simulink model "HybridFEMModel"  (Simulink 7.0)
settings: Solver=FixedStepDiscrete  SolverMode=SingleTasking  StartTime=0.0  StopTime=RunningTime  FixedStep=SampleRate  RelTol=1e-3
undefined symbols (not defined in the file): Alpham, DiscIntNeverNeededParam, Elements, gamma1, gamma2, sample, SampleRate
libraries: simulink x6
(part 3 of 4)

== system HybridFEMModel/Quad Ramp Gen AIC/inverse compensator ==
  note: dp
  note: d(alpha)
  note: dc
  In1 : Inport  OutDataType=sfix(16)  OutScaling=2^0
  In2 : Inport  Port=2  OutDataType=sfix(16)  OutScaling=2^0
  Discrete Transfer Fcn : DiscreteTransferFcn  Numerator=[1 -1]  Denominator=[1 0]  SampleTime=sample
  Product : Product  OutDataType=sfix(16)  OutScaling=2^0  RndMeth=Zero
  Scope : Scope
  Sum2 : Sum  Inputs=|++  OutDataType=sfix(16)  OutScaling=2^0
  Sum5 : Sum  Inputs=|++  OutDataType=sfix(16)  OutScaling=2^0
  Unit Delay : UnitDelay  SampleTime=sample
  alpham : Constant  Value=Alpham  OutDataType=sfix(16)  OutScaling=2^0
  Out1 : Outport  OutDataType=sfix(16)  OutScaling=2^0
  wires:
  Sum2/1 -> Out1/1
  Product/1 -> Sum2/2
  Unit Delay/1 -> Sum2/1
  Sum5/1 -> Scope/1, Product/2
  Discrete Transfer Fcn/1 -> Product/1
  alpham/1 -> Sum5/2
  In2/1 -> Sum5/1
  In1/1 -> Unit Delay/1, Discrete Transfer Fcn/1

== system HybridFEMModel/Linear AIC/Tracking Indicator/A ==
  note: TI
  note: dm
  note: dc
  In1 : Inport  OutDataType=sfix(16)  OutScaling=2^0
  In2 : Inport  Port=2  OutDataType=sfix(16)  OutScaling=2^0
  Gain : Gain  Gain=0.5  ParameterDataType=sfix(16)  ParameterScaling=2^0  OutDataType=sfix(16)  OutScaling=2^0
  Product1 : Product  OutDataType=sfix(16)  OutScaling=2^0  RndMeth=Zero
  Sum2 : Sum  Inputs=|++  OutDataType=sfix(16)  OutScaling=2^0
  Sum3 : Sum  Inputs=|+-  OutDataType=sfix(16)  OutScaling=2^0
  Unit Delay : UnitDelay  SampleTime=sample
  Unit Delay1 : UnitDelay  SampleTime=sample
  accumulation : DiscreteTransferFcn  Numerator=[1 0]  Denominator=[1 -1]  SampleTime=sample
  Out1 : Outport  OutDataType=sfix(16)  OutScaling=2^0
  wires:
  accumulation/1 -> Out1/1
  Gain/1 -> accumulation/1
  Product1/1 -> Gain/1
  Sum3/1 -> Product1/2
  Sum2/1 -> Product1/1
  Unit Delay1/1 -> Sum3/2
  Unit Delay/1 -> Sum2/1
  In2/1 -> Unit Delay1/1, Sum3/1
  In1/1 -> Sum2/2, Unit Delay/1

== system HybridFEMModel/Linear AIC/Tracking Indicator/TA ==
  note: TI
  note: dc
  note: dm
  In1 : Inport  OutDataType=sfix(16)  OutScaling=2^0
  In2 : Inport  Port=2  OutDataType=sfix(16)  OutScaling=2^0
  Gain : Gain  Gain=0.5  ParameterDataType=sfix(16)  ParameterScaling=2^0  OutDataType=sfix(16)  OutScaling=2^0
  Product1 : Product  OutDataType=sfix(16)  OutScaling=2^0  RndMeth=Zero
  Sum2 : Sum  Inputs=|++  OutDataType=sfix(16)  OutScaling=2^0
  Sum3 : Sum  Inputs=|+-  OutDataType=sfix(16)  OutScaling=2^0
  Unit Delay : UnitDelay  SampleTime=sample
  Unit Delay1 : UnitDelay  SampleTime=sample
  accumulation : DiscreteTransferFcn  Numerator=[1 0]  Denominator=[1 -1]  SampleTime=sample
  Out1 : Outport  OutDataType=sfix(16)  OutScaling=2^0
  wires:
  accumulation/1 -> Out1/1
  Gain/1 -> accumulation/1
  Product1/1 -> Gain/1
  Sum3/1 -> Product1/2
  Sum2/1 -> Product1/1
  Unit Delay1/1 -> Sum3/2
  Unit Delay/1 -> Sum2/1
  In1/1 -> Unit Delay1/1, Sum3/1
  In2/1 -> Sum2/2, Unit Delay/1

== system HybridFEMModel/Quad Ramp Gen AIC/Tracking Indicator/A ==
  note: dc
  note: dm
  note: TI
  In1 : Inport  OutDataType=sfix(16)  OutScaling=2^0
  In2 : Inport  Port=2  OutDataType=sfix(16)  OutScaling=2^0
  Gain : Gain  Gain=0.5  ParameterDataType=sfix(16)  ParameterScaling=2^0  OutDataType=sfix(16)  OutScaling=2^0
  Product1 : Product  OutDataType=sfix(16)  OutScaling=2^0  RndMeth=Zero
  Sum2 : Sum  Inputs=|++  OutDataType=sfix(16)  OutScaling=2^0
  Sum3 : Sum  Inputs=|+-  OutDataType=sfix(16)  OutScaling=2^0
  Unit Delay : UnitDelay  SampleTime=sample
  Unit Delay1 : UnitDelay  SampleTime=sample
  accumulation : DiscreteTransferFcn  Numerator=[1 0]  Denominator=[1 -1]  SampleTime=sample
  Out1 : Outport  OutDataType=sfix(16)  OutScaling=2^0
  wires:
  In1/1 -> Unit Delay/1, Sum2/2
  In2/1 -> Sum3/1, Unit Delay1/1
  Unit Delay/1 -> Sum2/1
  Unit Delay1/1 -> Sum3/2
  Sum2/1 -> Product1/1
  Sum3/1 -> Product1/2
  Product1/1 -> Gain/1
  Gain/1 -> accumulation/1
  accumulation/1 -> Out1/1

== system HybridFEMModel/Quad Ramp Gen AIC/Tracking Indicator/TA ==
  note: dm
  note: dc
  note: TI
  In1 : Inport  OutDataType=sfix(16)  OutScaling=2^0
  In2 : Inport  Port=2  OutDataType=sfix(16)  OutScaling=2^0
  Gain : Gain  Gain=0.5  ParameterDataType=sfix(16)  ParameterScaling=2^0  OutDataType=sfix(16)  OutScaling=2^0
  Product1 : Product  OutDataType=sfix(16)  OutScaling=2^0  RndMeth=Zero
  Sum2 : Sum  Inputs=|++  OutDataType=sfix(16)  OutScaling=2^0
  Sum3 : Sum  Inputs=|+-  OutDataType=sfix(16)  OutScaling=2^0
  Unit Delay : UnitDelay  SampleTime=sample
  Unit Delay1 : UnitDelay  SampleTime=sample
  accumulation : DiscreteTransferFcn  Numerator=[1 0]  Denominator=[1 -1]  SampleTime=sample
  Out1 : Outport  OutDataType=sfix(16)  OutScaling=2^0
  wires:
  In2/1 -> Unit Delay/1, Sum2/2
  In1/1 -> Sum3/1, Unit Delay1/1
  Unit Delay/1 -> Sum2/1
  Unit Delay1/1 -> Sum3/2
  Sum2/1 -> Product1/1
  Sum3/1 -> Product1/2
  Product1/1 -> Gain/1
  Gain/1 -> accumulation/1
  accumulation/1 -> Out1/1

== matlab function Generate Element Restoring Forces/Generate Type 2 Element Restoring Force/Type 2 Element RF ==
  data: Nodes output inherited; Element input inherited; RF output inherited; NumFreeDOF input inherited; Displacement input inherited; ActuatorRF input inherited
% get restoring force for the element
% returns (6x1) restoring force vector of element in global coordinates
function [Nodes,RF] = fcn(Element, NumFreeDOF, Displacement, ActuatorRF)

%% Simulation flag
simulation = 1;

%% Input mapping
Node1ID = Element(1);
Node2ID = Element(2);
Stiffness = Element(3);
Nodes = [Node1ID,Node2ID];

% Get distance between nodes
I1 = Node1ID;
I2 = Node2ID;

% preset arrays
SE = zeros(6,6);
    
% Form Stiffness Matrix
SE(1, 1) = Stiffness;
SE(1, 4) = -Stiffness;
SE(4, 4) = Stiffness;
SE(4, 1) = SE(1,4);

% Check if it is a simulation or using real RF
if (simulation == 1)
    %create the displacement Ue (6x1) vector of the element in global coordinates
    Ue = zeros(6, 1);
    if (I1 * 3) <= NumFreeDOF
        Ue(1, 1) = Displacement(I1 * 3 - 2, 1);
        Ue(2, 1) = Displacement(I1 * 3 - 1, 1);
        Ue(3, 1) = Displacement(I1 * 3, 1);
    end
    if (I2 * 3) <= NumFreeDOF
        Ue(4, 1) = Displacement(I2 * 3 - 2, 1);
        Ue(5, 1) = Displacement(I2 * 3 - 1, 1);
        Ue(6, 1) = Displacement(I2 * 3, 1);
    end
    RF = SE*Ue;  %resisting (6x1) resisting force vector of element in global coordinates
else
    RestoringForce = zeros(6,1);
    RestoringForce(1,1) = -ActuatorRF;
    RestoringForce(4,1) = ActuatorRF;
	RF = RestoringForce;
end

== matlab function Generate Element Restoring Forces/Form Total Restoring Force Vector/Form Restoring Force Vector ==
  data: Nodes_muxed input inherited; RF_muxed input inherited; TotalRF output inherited
function TotalRF = eml(Nodes_muxed,RF_muxed)
% This block supports the Embedded MATLAB subset.
% See the help menu for details. 

NumFreeDOF = 18;
TotalRF = zeros(NumFreeDOF,1);

for i = 2:2:length(Nodes_muxed)
    N1 = Nodes_muxed(i-1);
    N2 = Nodes_muxed(i);
    if (3 * N1) <= NumFreeDOF
        TotalRF(N1 * 3 - 2, 1) = RF_muxed(1+(6*(i-2)/2)) + TotalRF(N1 * 3 - 2, 1);
        TotalRF(N1 * 3 - 1, 1) = RF_muxed(2+(6*(i-2)/2)) + TotalRF(N1 * 3 - 1, 1);
        TotalRF(N1 * 3, 1) = RF_muxed(3+(6*(i-2)/2)) + TotalRF(N1 * 3, 1);
    end
    if (3 * N2) <= NumFreeDOF
        TotalRF(N2 * 3 - 2, 1) = RF_muxed(4+(6*(i-2)/2)) + TotalRF(N2 * 3 - 2, 1);
        TotalRF(N2 * 3 - 1, 1) = RF_muxed(5+(6*(i-2)/2)) + TotalRF(N2 * 3 - 1, 1);
        TotalRF(N2 * 3, 1) = RF_muxed(6+(6*(i-2)/2)) + TotalRF(N2 * 3, 1);
    end
end

== matlab function Generate Element Restoring Forces/Generate Type 3 Element Restoring Force1/Type 3 Element RF ==
  data: Nodes output inherited; Element input inherited; a1 input inherited; a2 input inherited; pmx input inherited; bmy_init input inherited; RF output inherited; NumFreeDOF input inherited; Displacement input inherited
% Get Restoring Force Type 3
function [Nodes,RF] = fnc(Element, a1, a2, pmx, bmy_init, NumFreeDOF, Displacement)

persistent initialized;
persistent kody;
persistent bmep;
persistent bmel;
persistent bmtot;
persistent bbmy;
persistent dpr;
persistent bmy;
persistent ftot;
persistent pracn;
persistent pracp;
persistent prtot;
persistent sftot;
persistent Uprev;

%% Input mapping
Node1ID = Element(1);
Node2ID = Element(2);
Nodes = [Node1ID,Node2ID];
ksurf = Element(3);
cosa = Element(4);
eal = Element(5);
ek11 = Element(6);
ek11h = Element(7);
ek12 = Element(8);
ek22 = Element(9);
ek22h = Element(10);
fl = Element(11);
pr12 = Element(12);
pr21 = Element(13);
psh = Element(14);
sina = Element(15);

if isempty(initialized)
    initialized = 1;
    kody = zeros(2,1);
    bmep = zeros(2,1); 
    bmel = zeros(2,1);
    bmtot = zeros(2,1);
    bbmy = 0;
    dpr = zeros(2,1);
    ftot = zeros(2,1);  
    pracn = zeros(2,1); 
    pracp = zeros(2,1);
    prtot = zeros(2,1);
    sftot = zeros(2,1); 
    Uprev = zeros(6,1);
    bmy = bmy_init;
end



%% Get distance between nodes
I1 = Node1ID; %Node1ID;
I2 = Node2ID; %Node2ID;

%% Get the displacement Ue (6x1) vector of the element in global coordinates
Ue = zeros(6,1);
if (I1 * 3) <= NumFreeDOF
    Ue(1, 1) = Displacement(I1 * 3 - 2, 1);
    Ue(2, 1) = Displacement(I1 * 3 - 1, 1);
    Ue(3, 1) = Displacement(I1 * 3, 1);
end
if (I2 * 3) <= NumFreeDOF
    Ue(4, 1) = Displacement(I2 * 3 - 2, 1);
    Ue(5, 1) = Displacement(I2 * 3 - 1, 1);
    Ue(6, 1) = Displacement(I2 * 3, 1);
end

%% Input of Drain State Determination Type 2 Element
ndof=6;  %the element has 6 dofs
ddise=Ue-Uprev;  %the incremental displacement vector ddise of the element in global coordinates 
Uprev=Ue; %update Uprev of element for use in next state determination call
%% calculate element deformation increments
[dvax,dvr] = ELDFO2(ddise,fl,cosa,sina);
%% UPDATE AXIAL FORCES AND AXIAL ENERGY
dfax=eal*dvax;      
ftot(1,1)=ftot(1,1)-dfax;
ftot(2,1)=ftot(2,1)+dfax;  
%% MOMENTS IN ELASTIC COMPONENT AT BEGINING OF STEP
bmel(1,1)=bmtot(1,1)-bmep(1,1);
bmel(2,1)=bmtot(2,1)-bmep(2,1);
%% LINEAR MOMENT INCREMENTS FOR ELASTO-PLASTIC COMPONENT - SET IN DBM
[dbm] = BMCAO2(dvr,kody,ek11,ek12,ek22,ek22h,ek11h);
%% TRACE NONLINEAR PATH FOR ELASTO-PLASTIC COMPONENT---state determination
facac=0.0;
while (facac<0.999999)
    factor=1.0-facac;
    % PLASTIC HINGE ROTATIONS
    kod=kody(1,1)+kody(2,1)-1.0;
    if(kod>0)
        % hinges at both ends
        dpr(1,1)=dvr(1,1);
        dpr(2,1)=dvr(2,1);
    elseif(kod==0)
        % hinge at one end only
        dpr(1,1)=dvr(1,1)+pr21*dvr(2,1);
        dpr(2,1)=dvr(2,1)+pr12*dvr(1,1);
    else
         %never executed
    end
         
    % CALCULATE WHICH END HAS NEXT EVENT IF YIELDS, SET KFAC=IEND AND BBMY=YIELD VALUE
    % SET EVENT FACTOR IN FACTOR
    kfac=3;
    for iend=1:2
        if (kody(iend,1)==0.0)
            dbmm=dbm(iend,1);
            % elastic, get factor for status change(no hinge at end)
            if (dbmm<0.0)
                dbmo=bmy(iend,2)-bmep(iend,1);
                if(dbmo>=dbmm) 
                    fac=dbmo/dbmm;
                else
                    fac=2.0;
                end 
                if (fac<=factor)
                    factor=fac;
                    bbmy=bmy(iend,2);
                    kfac=iend;
                end
            elseif(dbmm>0.0)
                dbmo=bmy(iend,1)-bmep(iend,1);
                if(dbmo<=dbmm) 
                    fac=dbmo/dbmm;
                else
                    fac=2.0;
                end 
                if (fac<=factor)
                    factor=fac;
                    bbmy=bmy(iend,1);
                    kfac=iend;
                end
            else
            end
        else
            % hinge at this end
            if(bmep(iend,1)*dpr(iend,1)<0.0)
            % unloading (plastic work negative)
                factor=0.0;
                kfac=0.0;
                kody(iend,1)=0.0;
            else
                % continuing to yield (plastic work positive)
            end
        end
    end
    % UPDATE BENDING STATE AND CALCULATE BENDING ENERGY
    % dbm= elastic increment - use if elastic bbmy= yield value - use if yields
    if(kfac~=0)
        for iend=1:2
            if(iend==kfac)
                % new hinge at this end
                bmep(iend,1)=bbmy;
                kody(iend,1)=1;
            elseif(kody(iend,1)==0)
                % this end remains elastic
                dmep=factor*dbm(iend,1);
                bmep(iend,1)=bmep(iend,1)+dmep;
            else
                % this end remains plastic
                dppr=factor*dpr(iend,1);
                prtot(iend,1)=prtot(iend,1)+dppr;
                if (dppr<0.0)
                    pracn(iend,1)=pracn(iend,1)+dppr;
                else
                    pracp(iend,1)=pracp(iend,1)+dppr;
                end
            end
        end
    else
        % unloads - factor=0.
    end
    % CHECK COMPLETION OF CYCLE
    facac=facac+factor;
    if (facac<0.99999)
        % cycle not completed, calculate new moment increments
        [dbm] = BMCAO2(dvr,kody,ek11,ek12,ek22,ek22h,ek11h);
    end
end
%% YIELD MOMENTS FOR NEXT STEP
if(ksurf==1)
    [bmy] = YMOM02(ftot,pmx,a1,a2,bmy);
    % CHECK YIELD SURFACE OVERSHOOT
    for iend=1:2
        if (kody(iend,1)~=0.0)
        % inelastic on old surface
            if (bmep(iend,1)>bmy(iend,1)) 
                % inelastic positive on new surface also
                bmep(iend,1)=bmy(iend,1);
            elseif (bmep(iend,1)<bmy(iend,2))
                % inelastic negative on new surface also
                bmep(iend,1)=bmy(iend,2);
            elseif ((bmep(iend,1)<(bmy(iend,1)*0.98)) && (bmep(iend,1)>(bmy(iend,2)*0.98)))
                % moves inside new surface by > 2% - reset yield code
                kody(iend,1)=0;
            else
            end
        else
            % elastic on old surface
            if (bmep(iend,1)>bmy(iend,1))
                % inelastic positive on new surface
                bmep(iend,1)=bmy(iend,1);
                kody(iend,1)=1;
            elseif (bmep(iend,1)<=bmy(iend,2))
                % inelastic negative on new surface
                bmep(iend,1)=bmy(iend,2);
                kody(iend,1)=1;
            else
            end
        end
    end
end
%% UPDATE TOTAL FORCES
dsf=(bmtot(1,1)+ bmtot(2,1))/fl;
ppsh=psh/(1.0-psh);
dmeli=(ek11*dvr(1,1)+ek12*dvr(2,1))*ppsh+bmel(1,1);
dmelj=(ek12*dvr(1,1)+ ek22*dvr(2,1))*ppsh+bmel(2,1);
bmtot(1,1)=bmep(1,1)+dmeli;
bmtot(2,1)=bmep(2,1)+dmelj;
dsf=dsf-(bmtot(1,1)+bmtot(2,1))/fl;
sftot(1,1)=sftot(1,1)-dsf;
sftot(2,1)=sftot(2,1)+dsf;

RF = ELASO2(ndof,ftot,cosa,sina,sftot,bmtot);





%%%%%%% FUNCTIONS %%%%%%%%%
function [bmy] = YMOM02(ftot,pmx,a1,a2,bmy)
facc=-1.0;
for iend = 1 : 2
    % Change sign of axial force and end 1
    fft = ftot(iend,1) * facc;
    facc = 1;
    fac = 1;
    for j = 1 : 2
        fac = -fac;
        yieldcalc = 0;  % flag if the yield moment is calculated inside 
                        % this next for loop
        for i = 1 : 3
            if (fft < pmx(i,j,iend))
                yieldcalc = 1;  % set flag since the condition was met
                % Calculate yield moment (M = a2 + a1P)
                bbmy = a2(i,j,iend) - a1(i,j,iend) * fft;
                if (fac * bbmy > 0) 
                    % Axial force is beyond Pc and Pt
                    bbmy = 0;
                end
                bmy(iend,j) = bbmy;
            end
        end
        % Only calculate yield moment if it wasn't calculated in the above
        % for loop
        if (yieldcalc == 0)
            i = 4;
            % Calculate yield moment (M = a2 + a1P)
            bbmy = a2(i,j,iend) - a1(i,j,iend) * fft;
            if (fac * bbmy > 0) 
                % Axial force is beyond Pc and Pt
                bbmy = 0;
            end
            bmy(iend,j) = bbmy;
        end
    end
end
%c ---------------------------------INTERCHANGE BMY(1,1) AND BMY(1,2) AND
%c ------------------------------AND ALSO CHANGE SIGN OF MOMENTS AT END 1
fac=-bmy(1,1);
bmy(1,1)=-bmy(1,2);
bmy(1,2)=fac;
      
      
      
      
      
function [dbm] = BMCAO2(dvr,kody,ek11,ek12,ek22,ek22h,ek11h)
dbm=zeros(2,1);
% c ------------------SET KYY TO INDICATE TYPE OF ELEMENT STIFFNESS TO USE
      kyy=kody(1,1)+2*kody(2,1)+1;
      if(kyy==1)
%c---no hinge at either end
        dbm(1,1)=ek11*dvr(1,1)+ek12*dvr(2,1);
        dbm(2,1)=ek12*dvr(1,1)+ek22*dvr(2,1);
      elseif(kyy==2)
%c---hinge at end 1
        dbm(1,1)=0.0;
        dbm(2,1)=ek22h*dvr(2,1);
      elseif(kyy==3)
%c---hinge at end 2
        dbm(1,1)=ek11h*dvr(1,1);
        dbm(2,1)=0.0;
      elseif(kyy==4)
%c---hinges at both end
        dbm(1,1)=0.0;
        dbm(2,1)=0.0;
       else
           %never executed
      end
      
      
      
      
      
      
      
      
      
      
   %%
function [relas] = ELASO2(ndof,ftot,cosa,sina,sftot,bmtot)
%%
relas=zeros(ndof,1);
%BASIC RESISTING FORCES
      relas(1,1)=(ftot(1,1)-0)*cosa-(sftot(1,1)-0)*sina;
      relas(2,1)=(ftot(1,1)-0)*sina+(sftot(1,1)-0)*cosa;
      relas(3,1)=bmtot(1,1)-0-0;
      relas(4,1)=(ftot(2,1)-0)*cosa-(sftot(2,1)-0)*sina;
      relas(5,1)=(ftot(2,1)-0)*sina+(sftot(2,1)-0)*cosa;
      relas(6,1)=bmtot(2,1)-0-0;
%%







%%
function [dvax,dvr] = ELDFO2(ddise,f1,cosa, sina) 
%%
dvr=zeros(2,1);
%DEFORMATION INCREMENTS OR DEFORMATION RATES
      dvax=cosa*(ddise(4,1)-ddise(1,1))+sina*(ddise(5,1)-ddise(2,1));
      rot=(sina*(ddise(4,1)-ddise(1,1))+cosa*(ddise(2,1)-ddise(5,1)))/f1;
      dvr(1,1)=ddise(3,1)+rot;
      dvr(2,1)=ddise(6,1)+rot;
%%

== matlab function Generate Element Restoring Forces/Generate Type 1 Element Restoring Force1/Type 1 Element RF ==
  data: Nodes output inherited; Element input inherited; RF output inherited; NumFreeDOF input inherited; Displacement input inherited
% get restoring force for the element
% returns (6x1) restoring force vector of element in global coordinates
function [Nodes,RF] = eml(Element, NumFreeDOF, Displacement)

%% Input mapping
Node1ID = Element(1);
Node1Xcoord = Element(2);
Node1Ycoord = Element(3);
Node2ID = Element(4);
Node2Xcoord = Element(5);
Node2Ycoord = Element(6);
MaterialE = Element(7);
Area = Element(8);
Inertia = Element(9);
Nodes = [Node1ID,Node2ID];

% Get distance between nodes
I1 = Node1ID;
I2 = Node2ID;
X21 = Node2Xcoord - Node1Xcoord;
Y21 = Node2Ycoord - Node1Ycoord;
EL = sqrt(X21 * X21 + Y21 * Y21);
EAL = MaterialE * Area / EL;
EIZL = MaterialE * Inertia / EL;
%calculation of density (the uniform load is only taken into account)
SEP = zeros(6);
SEP(1, 1) = EAL;
SEP(1, 4) = -EAL;
SEP(4, 4) = EAL;
SEP(2, 2) = 12 * EIZL / EL ^ 2;
SEP(2, 3) = 6 * EIZL / EL;
SEP(2, 5) = -SEP(2, 2);
SEP(2, 6) = SEP(2, 3);
SEP(3, 3) = 4 * EIZL;
SEP(3, 5) = -6 * EIZL / EL;
SEP(3, 6) = 2 * EIZL;
SEP(5, 5) = 12 * EIZL / EL ^ 2;
SEP(5, 6) = -6 * EIZL / EL;
SEP(6, 6) = 4 * EIZL;
for i = 1:6
   for j = i:6
      SEP(j, i) = SEP(i, j);
   end
end
DCOS = zeros(3,3);
DCOS(1, 1) = X21 / EL;
DCOS(1, 2) = Y21 / EL;
DCOS(1, 3) = 0;
DCOS(2, 1) = -DCOS(1, 2);
DCOS(2, 2) = DCOS(1, 1);
DCOS(2, 3) = 0;
DCOS(3, 1) = 0;
DCOS(3, 2) = 0;
DCOS(3, 3) = 1;
ALMBDA = zeros(6);       
for i = 1:2
   IK = 3 * (i - 1);
   for j = 1:3
      for k = 1:3
         ALMBDA(j + IK, k + IK) = DCOS(j, k);
      end
   end
end
SE = SEP * ALMBDA;
SEP = SE;
SE = ALMBDA' * SEP;
%create the displacement Ue (6x1) vector of the element in global coordinates
Ue = zeros(6,1);
if (I1 * 3) <= NumFreeDOF
    Ue(1, 1) = Displacement(I1 * 3 - 2, 1);
    Ue(2, 1) = Displacement(I1 * 3 - 1, 1);
    Ue(3, 1) = Displacement(I1 * 3, 1);
end
if (I2 * 3) <= NumFreeDOF
    Ue(4, 1) = Displacement(I2 * 3 - 2, 1);
    Ue(5, 1) = Displacement(I2 * 3 - 1, 1);
    Ue(6, 1) = Displacement(I2 * 3, 1);
end
RF = SE * Ue;  %resisting (6x1) resisting force vector of element in global coordinates

== matlab function Generate Element Restoring Forces/Generate Type 1 Element Restoring Force2/Type 1 Element RF ==
  data: Nodes output inherited; Element input inherited; RF output inherited; NumFreeDOF input inherited; Displacement input inherited
% get restoring force for the element
% returns (6x1) restoring force vector of element in global coordinates
function [Nodes,RF] = eml(Element, NumFreeDOF, Displacement)

%% Input mapping
Node1ID = Element(1);
Node1Xcoord = Element(2);
Node1Ycoord = Element(3);
Node2ID = Element(4);
Node2Xcoord = Element(5);
Node2Ycoord = Element(6);
MaterialE = Element(7);
Area = Element(8);
Inertia = Element(9);
Nodes = [Node1ID,Node2ID];

% Get distance between nodes
I1 = Node1ID;
I2 = Node2ID;
X21 = Node2Xcoord - Node1Xcoord;
Y21 = Node2Ycoord - Node1Ycoord;
EL = sqrt(X21 * X21 + Y21 * Y21);
EAL = MaterialE * Area / EL;
EIZL = MaterialE * Inertia / EL;
%calculation of density (the uniform load is only taken into account)
SEP = zeros(6);
SEP(1, 1) = EAL;
SEP(1, 4) = -EAL;
SEP(4, 4) = EAL;
SEP(2, 2) = 12 * EIZL / EL ^ 2;
SEP(2, 3) = 6 * EIZL / EL;
SEP(2, 5) = -SEP(2, 2);
SEP(2, 6) = SEP(2, 3);
SEP(3, 3) = 4 * EIZL;
SEP(3, 5) = -6 * EIZL / EL;
SEP(3, 6) = 2 * EIZL;
SEP(5, 5) = 12 * EIZL / EL ^ 2;
SEP(5, 6) = -6 * EIZL / EL;
SEP(6, 6) = 4 * EIZL;
for i = 1:6
   for j = i:6
      SEP(j, i) = SEP(i, j);
   end
end
DCOS = zeros(3,3);
DCOS(1, 1) = X21 / EL;
DCOS(1, 2) = Y21 / EL;
DCOS(1, 3) = 0;
DCOS(2, 1) = -DCOS(1, 2);
DCOS(2, 2) = DCOS(1, 1);
DCOS(2, 3) = 0;
DCOS(3, 1) = 0;
DCOS(3, 2) = 0;
DCOS(3, 3) = 1;
ALMBDA = zeros(6);       
for i = 1:2
   IK = 3 * (i - 1);
   for j = 1:3
      for k = 1:3
         ALMBDA(j + IK, k + IK) = DCOS(j, k);
      end
   end
end
SE = SEP * ALMBDA;
SEP = SE;
SE = ALMBDA' * SEP;
%create the displacement Ue (6x1) vector of the element in global coordinates
Ue = zeros(6,1);
if (I1 * 3) <= NumFreeDOF
    Ue(1, 1) = Displacement(I1 * 3 - 2, 1);
    Ue(2, 1) = Displacement(I1 * 3 - 1, 1);
    Ue(3, 1) = Displacement(I1 * 3, 1);
end
if (I2 * 3) <= NumFreeDOF
    Ue(4, 1) = Displacement(I2 * 3 - 2, 1);
    Ue(5, 1) = Displacement(I2 * 3 - 1, 1);
    Ue(6, 1) = Displacement(I2 * 3, 1);
end
RF = SE * Ue;  %resisting (6x1) resisting force vector of element in global coordinates

== matlab function Generate Element Restoring Forces/Generate Type 1 Element Restoring Force3/Type 1 Element RF ==
  data: Nodes output inherited; Element input inherited; RF output inherited; NumFreeDOF input inherited; Displacement input inherited
% get restoring force for the element
% returns (6x1) restoring force vector of element in global coordinates
function [Nodes,RF] = eml(Element, NumFreeDOF, Displacement)

%% Input mapping
Node1ID = Element(1);
Node1Xcoord = Element(2);
Node1Ycoord = Element(3);
Node2ID = Element(4);
Node2Xcoord = Element(5);
Node2Ycoord = Element(6);
MaterialE = Element(7);
Area = Element(8);
Inertia = Element(9);
Nodes = [Node1ID,Node2ID];

% Get distance between nodes
I1 = Node1ID;
I2 = Node2ID;
X21 = Node2Xcoord - Node1Xcoord;
Y21 = Node2Ycoord - Node1Ycoord;
EL = sqrt(X21 * X21 + Y21 * Y21);
EAL = MaterialE * Area / EL;
EIZL = MaterialE * Inertia / EL;
%calculation of density (the uniform load is only taken into account)
SEP = zeros(6);
SEP(1, 1) = EAL;
SEP(1, 4) = -EAL;
SEP(4, 4) = EAL;
SEP(2, 2) = 12 * EIZL / EL ^ 2;
SEP(2, 3) = 6 * EIZL / EL;
SEP(2, 5) = -SEP(2, 2);
SEP(2, 6) = SEP(2, 3);
SEP(3, 3) = 4 * EIZL;
SEP(3, 5) = -6 * EIZL / EL;
SEP(3, 6) = 2 * EIZL;
SEP(5, 5) = 12 * EIZL / EL ^ 2;
SEP(5, 6) = -6 * EIZL / EL;
SEP(6, 6) = 4 * EIZL;
for i = 1:6
   for j = i:6
      SEP(j, i) = SEP(i, j);
   end
end
DCOS = zeros(3,3);
DCOS(1, 1) = X21 / EL;
DCOS(1, 2) = Y21 / EL;
DCOS(1, 3) = 0;
DCOS(2, 1) = -DCOS(1, 2);
DCOS(2, 2) = DCOS(1, 1);
DCOS(2, 3) = 0;
DCOS(3, 1) = 0;
DCOS(3, 2) = 0;
DCOS(3, 3) = 1;
ALMBDA = zeros(6);       
for i = 1:2
   IK = 3 * (i - 1);
   for j = 1:3
      for k = 1:3
         ALMBDA(j + IK, k + IK) = DCOS(j, k);
      end
   end
end
SE = SEP * ALMBDA;
SEP = SE;
SE = ALMBDA' * SEP;
%create the displacement Ue (6x1) vector of the element in global coordinates
Ue = zeros(6,1);
if (I1 * 3) <= NumFreeDOF
    Ue(1, 1) = Displacement(I1 * 3 - 2, 1);
    Ue(2, 1) = Displacement(I1 * 3 - 1, 1);
    Ue(3, 1) = Displacement(I1 * 3, 1);
end
if (I2 * 3) <= NumFreeDOF
    Ue(4, 1) = Displacement(I2 * 3 - 2, 1);
    Ue(5, 1) = Displacement(I2 * 3 - 1, 1);
    Ue(6, 1) = Displacement(I2 * 3, 1);
end
RF = SE * Ue;  %resisting (6x1) resisting force vector of element in global coordinates

== matlab function Generate Element Restoring Forces/Generate Type 1 Element Restoring Force4/Type 1 Element RF ==
  data: Nodes output inherited; Element input inherited; RF output inherited; NumFreeDOF input inherited; Displacement input inherited
% get restoring force for the element
% returns (6x1) restoring force vector of element in global coordinates
function [Nodes,RF] = eml(Element, NumFreeDOF, Displacement)

%% Input mapping
Node1ID = Element(1);
Node1Xcoord = Element(2);
Node1Ycoord = Element(3);
Node2ID = Element(4);
Node2Xcoord = Element(5);
Node2Ycoord = Element(6);
MaterialE = Element(7);
Area = Element(8);
Inertia = Element(9);
Nodes = [Node1ID,Node2ID];

% Get distance between nodes
I1 = Node1ID;
I2 = Node2ID;
X21 = Node2Xcoord - Node1Xcoord;
Y21 = Node2Ycoord - Node1Ycoord;
EL = sqrt(X21 * X21 + Y21 * Y21);
EAL = MaterialE * Area / EL;
EIZL = MaterialE * Inertia / EL;
%calculation of density (the uniform load is only taken into account)
SEP = zeros(6);
SEP(1, 1) = EAL;
SEP(1, 4) = -EAL;
SEP(4, 4) = EAL;
SEP(2, 2) = 12 * EIZL / EL ^ 2;
SEP(2, 3) = 6 * EIZL / EL;
SEP(2, 5) = -SEP(2, 2);
SEP(2, 6) = SEP(2, 3);
SEP(3, 3) = 4 * EIZL;
SEP(3, 5) = -6 * EIZL / EL;
SEP(3, 6) = 2 * EIZL;
SEP(5, 5) = 12 * EIZL / EL ^ 2;
SEP(5, 6) = -6 * EIZL / EL;
SEP(6, 6) = 4 * EIZL;
for i = 1:6
   for j = i:6
      SEP(j, i) = SEP(i, j);
   end
end
DCOS = zeros(3,3);
DCOS(1, 1) = X21 / EL;
DCOS(1, 2) = Y21 / EL;
DCOS(1, 3) = 0;
DCOS(2, 1) = -DCOS(1, 2);
DCOS(2, 2) = DCOS(1, 1);
DCOS(2, 3) = 0;
DCOS(3, 1) = 0;
DCOS(3, 2) = 0;
DCOS(3, 3) = 1;
ALMBDA = zeros(6);       
for i = 1:2
   IK = 3 * (i - 1);
   for j = 1:3
      for k = 1:3
         ALMBDA(j + IK, k + IK) = DCOS(j, k);
      end
   end
end
SE = SEP * ALMBDA;
SEP = SE;
SE = ALMBDA' * SEP;
%create the displacement Ue (6x1) vector of the element in global coordinates
Ue = zeros(6,1);
if (I1 * 3) <= NumFreeDOF
    Ue(1, 1) = Displacement(I1 * 3 - 2, 1);
    Ue(2, 1) = Displacement(I1 * 3 - 1, 1);
    Ue(3, 1) = Displacement(I1 * 3, 1);
end
if (I2 * 3) <= NumFreeDOF
    Ue(4, 1) = Displacement(I2 * 3 - 2, 1);
    Ue(5, 1) = Displacement(I2 * 3 - 1, 1);
    Ue(6, 1) = Displacement(I2 * 3, 1);
end
RF = SE * Ue;  %resisting (6x1) resisting force vector of element in global coordinates

== matlab function Generate Element Restoring Forces/Generate Type 1 Element Restoring Force5/Type 1 Element RF ==
  data: Nodes output inherited; Element input inherited; RF output inherited; NumFreeDOF input inherited; Displacement input inherited
% get restoring force for the element
% returns (6x1) restoring force vector of element in global coordinates
function [Nodes,RF] = eml(Element, NumFreeDOF, Displacement)

%% Input mapping
Node1ID = Element(1);
Node1Xcoord = Element(2);
Node1Ycoord = Element(3);
Node2ID = Element(4);
Node2Xcoord = Element(5);
Node2Ycoord = Element(6);
MaterialE = Element(7);
Area = Element(8);
Inertia = Element(9);
Nodes = [Node1ID,Node2ID];

% Get distance between nodes
I1 = Node1ID;
I2 = Node2ID;
X21 = Node2Xcoord - Node1Xcoord;
Y21 = Node2Ycoord - Node1Ycoord;
EL = sqrt(X21 * X21 + Y21 * Y21);
EAL = MaterialE * Area / EL;
EIZL = MaterialE * Inertia / EL;
%calculation of density (the uniform load is only taken into account)
SEP = zeros(6);
SEP(1, 1) = EAL;
SEP(1, 4) = -EAL;
SEP(4, 4) = EAL;
SEP(2, 2) = 12 * EIZL / EL ^ 2;
SEP(2, 3) = 6 * EIZL / EL;
SEP(2, 5) = -SEP(2, 2);
SEP(2, 6) = SEP(2, 3);
SEP(3, 3) = 4 * EIZL;
SEP(3, 5) = -6 * EIZL / EL;
SEP(3, 6) = 2 * EIZL;
SEP(5, 5) = 12 * EIZL / EL ^ 2;
SEP(5, 6) = -6 * EIZL / EL;
SEP(6, 6) = 4 * EIZL;
for i = 1:6
   for j = i:6
      SEP(j, i) = SEP(i, j);
   end
end
DCOS = zeros(3,3);
DCOS(1, 1) = X21 / EL;
DCOS(1, 2) = Y21 / EL;
DCOS(1, 3) = 0;
DCOS(2, 1) = -DCOS(1, 2);
DCOS(2, 2) = DCOS(1, 1);
DCOS(2, 3) = 0;
DCOS(3, 1) = 0;
DCOS(3, 2) = 0;
DCOS(3, 3) = 1;
ALMBDA = zeros(6);       
for i = 1:2
   IK = 3 * (i - 1);
   for j = 1:3
      for k = 1:3
         ALMBDA(j + IK, k + IK) = DCOS(j, k);
      end
   end
end
SE = SEP * ALMBDA;
SEP = SE;
SE = ALMBDA' * SEP;
%create the displacement Ue (6x1) vector of the element in global coordinates
Ue = zeros(6,1);
if (I1 * 3) <= NumFreeDOF
    Ue(1, 1) = Displacement(I1 * 3 - 2, 1);
    Ue(2, 1) = Displacement(I1 * 3 - 1, 1);
    Ue(3, 1) = Displacement(I1 * 3, 1);
end
if (I2 * 3) <= NumFreeDOF
    Ue(4, 1) = Displacement(I2 * 3 - 2, 1);
    Ue(5, 1) = Displacement(I2 * 3 - 1, 1);
    Ue(6, 1) = Displacement(I2 * 3, 1);
end
RF = SE * Ue;  %resisting (6x1) resisting force vector of element in global coordinates

== matlab function Generate Element Restoring Forces/Generate Type 3 Element Restoring Force/Type 3 Element RF ==
  data: Nodes output inherited; Element input inherited; a1 input inherited; a2 input inherited; pmx input inherited; bmy_init input inherited; RF output inherited; NumFreeDOF input inherited; Displacement input inherited
% Get Restoring Force Type 3
function [Nodes,RF] = fnc(Element, a1, a2, pmx, bmy_init, NumFreeDOF, Displacement)

persistent initialized;
persistent kody;
persistent bmep;
persistent bmel;
persistent bmtot;
persistent bbmy;
persistent dpr;
persistent bmy;
persistent ftot;
persistent pracn;
persistent pracp;
persistent prtot;
persistent sftot;
persistent Uprev;

%% Input mapping
Node1ID = Element(1);
Node2ID = Element(2);
Nodes = [Node1ID,Node2ID];
ksurf = Element(3);
cosa = Element(4);
eal = Element(5);
ek11 = Element(6);
ek11h = Element(7);
ek12 = Element(8);
ek22 = Element(9);
ek22h = Element(10);
fl = Element(11);
pr12 = Element(12);
pr21 = Element(13);
psh = Element(14);
sina = Element(15);

if isempty(initialized)
    initialized = 1;
    kody = zeros(2,1);
    bmep = zeros(2,1); 
    bmel = zeros(2,1);
    bmtot = zeros(2,1);
    bbmy = 0;
    dpr = zeros(2,1);
    ftot = zeros(2,1);  
    pracn = zeros(2,1); 
    pracp = zeros(2,1);
    prtot = zeros(2,1);
    sftot = zeros(2,1); 
    Uprev = zeros(6,1);
    bmy = bmy_init;
end



%% Get distance between nodes
I1 = Node1ID; %Node1ID;
I2 = Node2ID; %Node2ID;

%% Get the displacement Ue (6x1) vector of the element in global coordinates
Ue = zeros(6,1);
if (I1 * 3) <= NumFreeDOF
    Ue(1, 1) = Displacement(I1 * 3 - 2, 1);
    Ue(2, 1) = Displacement(I1 * 3 - 1, 1);
    Ue(3, 1) = Displacement(I1 * 3, 1);
end
if (I2 * 3) <= NumFreeDOF
    Ue(4, 1) = Displacement(I2 * 3 - 2, 1);
    Ue(5, 1) = Displacement(I2 * 3 - 1, 1);
    Ue(6, 1) = Displacement(I2 * 3, 1);
end

%% Input of Drain State Determination Type 2 Element
ndof=6;  %the element has 6 dofs
ddise=Ue-Uprev;  %the incremental displacement vector ddise of the element in global coordinates 
Uprev=Ue; %update Uprev of element for use in next state determination call
%% calculate element deformation increments
[dvax,dvr] = ELDFO2(ddise,fl,cosa,sina);
%% UPDATE AXIAL FORCES AND AXIAL ENERGY
dfax=eal*dvax;      
ftot(1,1)=ftot(1,1)-dfax;
ftot(2,1)=ftot(2,1)+dfax;  
%% MOMENTS IN ELASTIC COMPONENT AT BEGINING OF STEP
bmel(1,1)=bmtot(1,1)-bmep(1,1);
bmel(2,1)=bmtot(2,1)-bmep(2,1);
%% LINEAR MOMENT INCREMENTS FOR ELASTO-PLASTIC COMPONENT - SET IN DBM
[dbm] = BMCAO2(dvr,kody,ek11,ek12,ek22,ek22h,ek11h);
%% TRACE NONLINEAR PATH FOR ELASTO-PLASTIC COMPONENT---state determination
facac=0.0;
while (facac<0.999999)
    factor=1.0-facac;
    % PLASTIC HINGE ROTATIONS
    kod=kody(1,1)+kody(2,1)-1.0;
    if(kod>0)
        % hinges at both ends
        dpr(1,1)=dvr(1,1);
        dpr(2,1)=dvr(2,1);
    elseif(kod==0)
        % hinge at one end only
        dpr(1,1)=dvr(1,1)+pr21*dvr(2,1);
        dpr(2,1)=dvr(2,1)+pr12*dvr(1,1);
    else
         %never executed
    end
         
    % CALCULATE WHICH END HAS NEXT EVENT IF YIELDS, SET KFAC=IEND AND BBMY=YIELD VALUE
    % SET EVENT FACTOR IN FACTOR
    kfac=3;
    for iend=1:2
        if (kody(iend,1)==0.0)
            dbmm=dbm(iend,1);
            % elastic, get factor for status change(no hinge at end)
            if (dbmm<0.0)
                dbmo=bmy(iend,2)-bmep(iend,1);
                if(dbmo>=dbmm) 
                    fac=dbmo/dbmm;
                else
                    fac=2.0;
                end 
                if (fac<=factor)
                    factor=fac;
                    bbmy=bmy(iend,2);
                    kfac=iend;
                end
            elseif(dbmm>0.0)
                dbmo=bmy(iend,1)-bmep(iend,1);
                if(dbmo<=dbmm) 
                    fac=dbmo/dbmm;
                else
                    fac=2.0;
                end 
                if (fac<=factor)
                    factor=fac;
                    bbmy=bmy(iend,1);
                    kfac=iend;
                end
            else
            end
        else
            % hinge at this end
            if(bmep(iend,1)*dpr(iend,1)<0.0)
            % unloading (plastic work negative)
                factor=0.0;
                kfac=0.0;
                kody(iend,1)=0.0;
            else
                % continuing to yield (plastic work positive)
            end
        end
    end
    % UPDATE BENDING STATE AND CALCULATE BENDING ENERGY
    % dbm= elastic increment - use if elastic bbmy= yield value - use if yields
    if(kfac~=0)
        for iend=1:2
            if(iend==kfac)
                % new hinge at this end
                bmep(iend,1)=bbmy;
                kody(iend,1)=1;
            elseif(kody(iend,1)==0)
                % this end remains elastic
                dmep=factor*dbm(iend,1);
                bmep(iend,1)=bmep(iend,1)+dmep;
            else
                % this end remains plastic
                dppr=factor*dpr(iend,1);
                prtot(iend,1)=prtot(iend,1)+dppr;
                if (dppr<0.0)
                    pracn(iend,1)=pracn(iend,1)+dppr;
                else
                    pracp(iend,1)=pracp(iend,1)+dppr;
                end
            end
        end
    else
        % unloads - factor=0.
    end
    % CHECK COMPLETION OF CYCLE
    facac=facac+factor;
    if (facac<0.99999)
        % cycle not completed, calculate new moment increments
        [dbm] = BMCAO2(dvr,kody,ek11,ek12,ek22,ek22h,ek11h);
    end
end
%% YIELD MOMENTS FOR NEXT STEP
if(ksurf==1)
    [bmy] = YMOM02(ftot,pmx,a1,a2,bmy);
    % CHECK YIELD SURFACE OVERSHOOT
    for iend=1:2
        if (kody(iend,1)~=0.0)
        % inelastic on old surface
            if (bmep(iend,1)>bmy(iend,1)) 
                % inelastic positive on new surface also
                bmep(iend,1)=bmy(iend,1);
            elseif (bmep(iend,1)<bmy(iend,2))
                % inelastic negative on new surface also
                bmep(iend,1)=bmy(iend,2);
            elseif ((bmep(iend,1)<(bmy(iend,1)*0.98)) && (bmep(iend,1)>(bmy(iend,2)*0.98)))
                % moves inside new surface by > 2% - reset yield code
                kody(iend,1)=0;
            else
            end
        else
            % elastic on old surface
            if (bmep(iend,1)>bmy(iend,1))
                % inelastic positive on new surface
                bmep(iend,1)=bmy(iend,1);
                kody(iend,1)=1;
            elseif (bmep(iend,1)<=bmy(iend,2))
                % inelastic negative on new surface
                bmep(iend,1)=bmy(iend,2);
                kody(iend,1)=1;
            else
            end
        end
    end
end
%% UPDATE TOTAL FORCES
dsf=(bmtot(1,1)+ bmtot(2,1))/fl;
ppsh=psh/(1.0-psh);
dmeli=(ek11*dvr(1,1)+ek12*dvr(2,1))*ppsh+bmel(1,1);
dmelj=(ek12*dvr(1,1)+ ek22*dvr(2,1))*ppsh+bmel(2,1);
bmtot(1,1)=bmep(1,1)+dmeli;
bmtot(2,1)=bmep(2,1)+dmelj;
dsf=dsf-(bmtot(1,1)+bmtot(2,1))/fl;
sftot(1,1)=sftot(1,1)-dsf;
sftot(2,1)=sftot(2,1)+dsf;

RF = ELASO2(ndof,ftot,cosa,sina,sftot,bmtot);





%%%%%%% FUNCTIONS %%%%%%%%%
function [bmy] = YMOM02(ftot,pmx,a1,a2,bmy)
facc=-1.0;
for iend = 1 : 2
    % Change sign of axial force and end 1
    fft = ftot(iend,1) * facc;
    facc = 1;
    fac = 1;
    for j = 1 : 2
        fac = -fac;
        yieldcalc = 0;  % flag if the yield moment is calculated inside 
                        % this next for loop
        for i = 1 : 3
            if (fft < pmx(i,j,iend))
                yieldcalc = 1;  % set flag since the condition was met
                % Calculate yield moment (M = a2 + a1P)
                bbmy = a2(i,j,iend) - a1(i,j,iend) * fft;
                if (fac * bbmy > 0) 
                    % Axial force is beyond Pc and Pt
                    bbmy = 0;
                end
                bmy(iend,j) = bbmy;
            end
        end
        % Only calculate yield moment if it wasn't calculated in the above
        % for loop
        if (yieldcalc == 0)
            i = 4;
            % Calculate yield moment (M = a2 + a1P)
            bbmy = a2(i,j,iend) - a1(i,j,iend) * fft;
            if (fac * bbmy > 0) 
                % Axial force is beyond Pc and Pt
                bbmy = 0;
            end
            bmy(iend,j) = bbmy;
        end
    end
end
%c ---------------------------------INTERCHANGE BMY(1,1) AND BMY(1,2) AND
%c ------------------------------AND ALSO CHANGE SIGN OF MOMENTS AT END 1
fac=-bmy(1,1);
bmy(1,1)=-bmy(1,2);
bmy(1,2)=fac;
      
      
      
      
      
function [dbm] = BMCAO2(dvr,kody,ek11,ek12,ek22,ek22h,ek11h)
dbm=zeros(2,1);
% c ------------------SET KYY TO INDICATE TYPE OF ELEMENT STIFFNESS TO USE
      kyy=kody(1,1)+2*kody(2,1)+1;
      if(kyy==1)
%c---no hinge at either end
        dbm(1,1)=ek11*dvr(1,1)+ek12*dvr(2,1);
        dbm(2,1)=ek12*dvr(1,1)+ek22*dvr(2,1);
      elseif(kyy==2)
%c---hinge at end 1
        dbm(1,1)=0.0;
        dbm(2,1)=ek22h*dvr(2,1);
      elseif(kyy==3)
%c---hinge at end 2
        dbm(1,1)=ek11h*dvr(1,1);
        dbm(2,1)=0.0;
      elseif(kyy==4)
%c---hinges at both end
        dbm(1,1)=0.0;
        dbm(2,1)=0.0;
       else
           %never executed
      end
      
      
      
      
      
      
      
      
      
      
   %%
function [relas] = ELASO2(ndof,ftot,cosa,sina,sftot,bmtot)
%%
relas=zeros(ndof,1);
%BASIC RESISTING FORCES
      relas(1,1)=(ftot(1,1)-0)*cosa-(sftot(1,1)-0)*sina;
      relas(2,1)=(ftot(1,1)-0)*sina+(sftot(1,1)-0)*cosa;
      relas(3,1)=bmtot(1,1)-0-0;
      relas(4,1)=(ftot(2,1)-0)*cosa-(sftot(2,1)-0)*sina;
      relas(5,1)=(ftot(2,1)-0)*sina+(sftot(2,1)-0)*cosa;
      relas(6,1)=bmtot(2,1)-0-0;
%%







%%
function [dvax,dvr] = ELDFO2(ddise,f1,cosa, sina) 
%%
dvr=zeros(2,1);
%DEFORMATION INCREMENTS OR DEFORMATION RATES
      dvax=cosa*(ddise(4,1)-ddise(1,1))+sina*(ddise(5,1)-ddise(2,1));
      rot=(sina*(ddise(4,1)-ddise(1,1))+cosa*(ddise(2,1)-ddise(5,1)))/f1;
      dvr(1,1)=ddise(3,1)+rot;
      dvr(2,1)=ddise(6,1)+rot;
%%

== matlab function Generate Acceleration Vector/Generate Acceleration Vector ==
  data: TotalRF input inherited; PEFF input inherited; M_FreeInv input inherited; Acceleration output inherited; C_Free input inherited; Velocity input inherited; step_count input inherited
function Acceleration = eml(TotalRF,PEFF,M_FreeInv,C_Free,Velocity,step_count)
% This block supports the Embedded MATLAB subset.
% See the help menu for details. 

Acceleration = M_FreeInv * (PEFF(step_count,:)' - C_Free * Velocity - TotalRF);

== matlab function Generate Command Vectors/Generate Command Vectors ==
  data: Timestep input inherited; Displacement_v output inherited; Beta1 input inherited; Beta2 input inherited; Displacement input inherited; Velocity input inherited; Acceleration input inherited; Velocity_v output inherited
function [Displacement_v,Velocity_v] = eml(Timestep, Beta1, Beta2, Displacement, Velocity, Acceleration)
% This block supports the Embedded MATLAB subset.
% See the help menu for details. 

Displacement_v = Displacement + Timestep*Velocity + Beta2*Timestep^2*Acceleration;
Velocity_v = Velocity + Beta1*Timestep*Acceleration;
